simulink model "VLDO_Simscape_test_no_graphs"  (R2016a)
settings: Solver=ode15s  StartTime=0.0  StopTime=5790*3  MaxStep=0.1  RelTol=1e-3
libraries: nesl_utility x38, fl_lib x36, elec_lib x15, simulink x1
(part 2 of 2)

== system VLDO_Simscape_test_no_graphs/ Load/Current Sensor (Load)2 ==
  Current Sensor : fl_lib/Electrical/Electrical Sensors/Current Sensor
  PS-Simulink : nesl_utility/PS-Simulink Converter  PhysicalDomain=network_engine_domain  SubClassName=ps_output  LeftPortType=input  RightPortType=output  PseudoPeriodic=off  Frequencies=[]  Unit=A  AffineConversion=off
  + : PMIOPort  Port=1  Side=Left
  - : PMIOPort  Port=2  Side=Left
  i : Outport
  wires:
  PS-Simulink/1 -> i/1
  connections:
  -/RConn1 -- Current Sensor/RConn2
  +/RConn1 -- Current Sensor/LConn1
  Current Sensor/RConn1 -- PS-Simulink/LConn1

== system VLDO_Simscape_test_no_graphs/ Load/Voltage Sensor (Diode)1 ==
  PS-Simulink : nesl_utility/PS-Simulink Converter  PhysicalDomain=network_engine_domain  SubClassName=ps_output  LeftPortType=input  RightPortType=output  PseudoPeriodic=off  Frequencies=[]  Unit=V  AffineConversion=off
  Voltage Sensor : fl_lib/Electrical/Electrical Sensors/Voltage Sensor
  + : PMIOPort  Port=1  Side=Left
  - : PMIOPort  Port=2  Side=Left
  v : Outport
  wires:
  PS-Simulink/1 -> v/1
  connections:
  -/RConn1 -- Voltage Sensor/RConn2
  +/RConn1 -- Voltage Sensor/LConn1
  Voltage Sensor/RConn1 -- PS-Simulink/LConn1

== system VLDO_Simscape_test_no_graphs/ Load/Voltage Sensor (Diode)4 ==
  PS-Simulink : nesl_utility/PS-Simulink Converter  PhysicalDomain=network_engine_domain  SubClassName=ps_output  LeftPortType=input  RightPortType=output  PseudoPeriodic=off  Frequencies=[]  Unit=V  AffineConversion=off
  Voltage Sensor : fl_lib/Electrical/Electrical Sensors/Voltage Sensor
  + : PMIOPort  Port=1  Side=Left
  - : PMIOPort  Port=2  Side=Left
  v : Outport
  wires:
  PS-Simulink/1 -> v/1
  connections:
  -/RConn1 -- Voltage Sensor/RConn2
  +/RConn1 -- Voltage Sensor/LConn1
  Voltage Sensor/RConn1 -- PS-Simulink/LConn1

== system VLDO_Simscape_test_no_graphs/Solar Panel 1/If Action Subsystem ==
  In1 : Inport
  In2 : Inport  Port=2
  Action Port : ActionPort  ActionType=then
  Out1 : Outport
  Out2 : Outport  Port=2
  wires:
  In1/1 -> Out1/1
  In2/1 -> Out2/1

== system VLDO_Simscape_test_no_graphs/Solar Panel 1/If Action Subsystem1 ==
  In1 : Inport
  In2 : Inport  Port=2
  Action Port : ActionPort  ActionType=elseif
  Out1 : Outport
  Out2 : Outport  Port=2
  wires:
  In1/1 -> Out1/1
  In2/1 -> Out2/1

== system VLDO_Simscape_test_no_graphs/Solar Panel 1/If Action Subsystem2 ==
  In1 : Inport
  In2 : Inport  Port=2
  Action Port : ActionPort  ActionType=else
  Out1 : Outport
  Out2 : Outport  Port=2
  wires:
  In1/1 -> Out1/1
  In2/1 -> Out2/1

== system VLDO_Simscape_test_no_graphs/Solar Panel 2/If Action Subsystem ==
  In1 : Inport
  In2 : Inport  Port=2
  Action Port : ActionPort  ActionType=then
  Out1 : Outport
  Out2 : Outport  Port=2
  wires:
  In1/1 -> Out1/1
  In2/1 -> Out2/1

== system VLDO_Simscape_test_no_graphs/Solar Panel 2/If Action Subsystem1 ==
  In1 : Inport
  In2 : Inport  Port=2
  Action Port : ActionPort  ActionType=elseif
  Out1 : Outport
  Out2 : Outport  Port=2
  wires:
  In1/1 -> Out1/1
  In2/1 -> Out2/1

== system VLDO_Simscape_test_no_graphs/Solar Panel 2/If Action Subsystem2 ==
  In1 : Inport
  In2 : Inport  Port=2
  Action Port : ActionPort  ActionType=else
  Out1 : Outport
  Out2 : Outport  Port=2
  wires:
  In1/1 -> Out1/1
  In2/1 -> Out2/1

== system VLDO_Simscape_test_no_graphs/Solar Panel 3/If Action Subsystem ==
  In1 : Inport
  In2 : Inport  Port=2
  Action Port : ActionPort  ActionType=then
  Out1 : Outport
  Out2 : Outport  Port=2
  wires:
  In1/1 -> Out1/1
  In2/1 -> Out2/1

== system VLDO_Simscape_test_no_graphs/Solar Panel 3/If Action Subsystem1 ==
  In1 : Inport
  In2 : Inport  Port=2
  Action Port : ActionPort  ActionType=elseif
  Out1 : Outport
  Out2 : Outport  Port=2
  wires:
  In1/1 -> Out1/1
  In2/1 -> Out2/1

== system VLDO_Simscape_test_no_graphs/Solar Panel 3/If Action Subsystem2 ==
  In1 : Inport
  In2 : Inport  Port=2
  Action Port : ActionPort  ActionType=else
  Out1 : Outport
  Out2 : Outport  Port=2
  wires:
  In1/1 -> Out1/1
  In2/1 -> Out2/1
